simulink model "rtwdemo_relationalsl"  (Simulink 7.1)
settings: Solver=FixedStepDiscrete  StartTime=0.0  StopTime=10.0  RelTol=1e-3
settings Model: Creator=ajayaram  LastModifiedBy=ajayaram
settings OptimizationCC: InlineParams=on  OptimizeModelRefInitCode=on  LifeSpan=1
settings RTWCC: SystemTargetFile=ert.tlc  GenerateMakefile=off  TemplateMakefile=ert_default_tmf  Description=Real-Time Workshop Embedded Coder (no auto configuration)  GenerateReport=on  ProcessScript=ert_make_rtw_hook  IncludeHyperlinkInReport=on  LaunchReport=on
settings CodeAppCC: GenerateComments=off  IgnoreCustomStorageClasses=off  SimulinkBlockComments=off
settings ERTTargetCC: GenerateSampleERTMain=on  InlinedParameterPlacement=NonHierarchical  ERTCustomFileTemplate=example_file_process.tlc

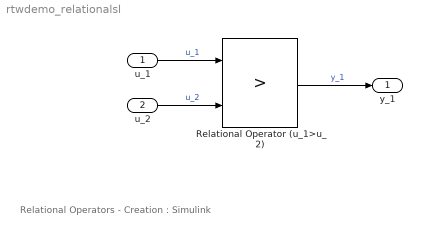
== system rtwdemo_relationalsl ==
  note: Relational Operators - Creation : Simulink
  u_1 : Inport  DataType=int16  OutDataType=sfix(16)  OutScaling=2^0  OutDataTypeStr=int16
  u_2 : Inport  Port=2  DataType=int16  OutDataType=sfix(16)  OutScaling=2^0  OutDataTypeStr=int16
  Relational Operator (u_1>u_2) : RelationalOperator  Operator=>  LogicOutDataTypeMode=boolean  OutDataTypeStr=boolean
  y_1 : Outport  OutDataType=sfix(16)  OutScaling=2^0
  wires:
  u_1/1 -> Relational Operator (u_1>u_2)/1  "u_1"
  u_2/1 -> Relational Operator (u_1>u_2)/2  "u_2"
  Relational Operator (u_1>u_2)/1 -> y_1/1  "y_1"
